simulink library "DLE_position_controller_v2"  (R2025b)
settings: Solver=VariableStepAuto  StartTime=0.0  StopTime=10.0  RelTol=1e-3
libraries: simulink x4, slpidlib x3, eeGeneralControl x1, dspstat3 x1
settings Model: Creator=cmmcguir  LastModifiedBy=cmmcguir

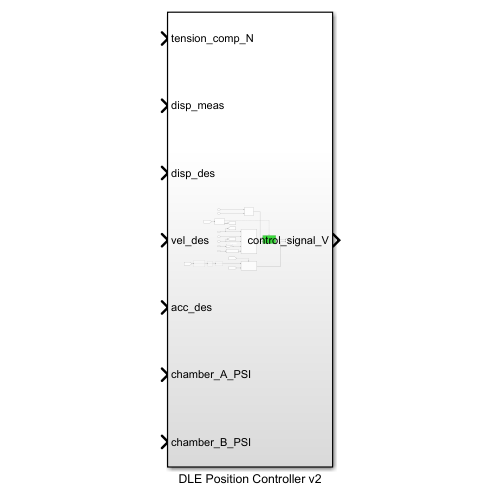
[thumbnail: Simulink's stored preview of the top-level diagram]
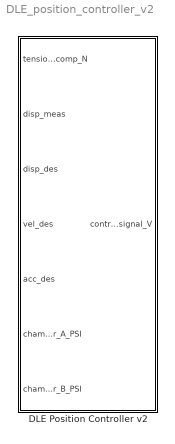
== system DLE_position_controller_v2 ==
  DLE Position Controller v2 : Subsystem

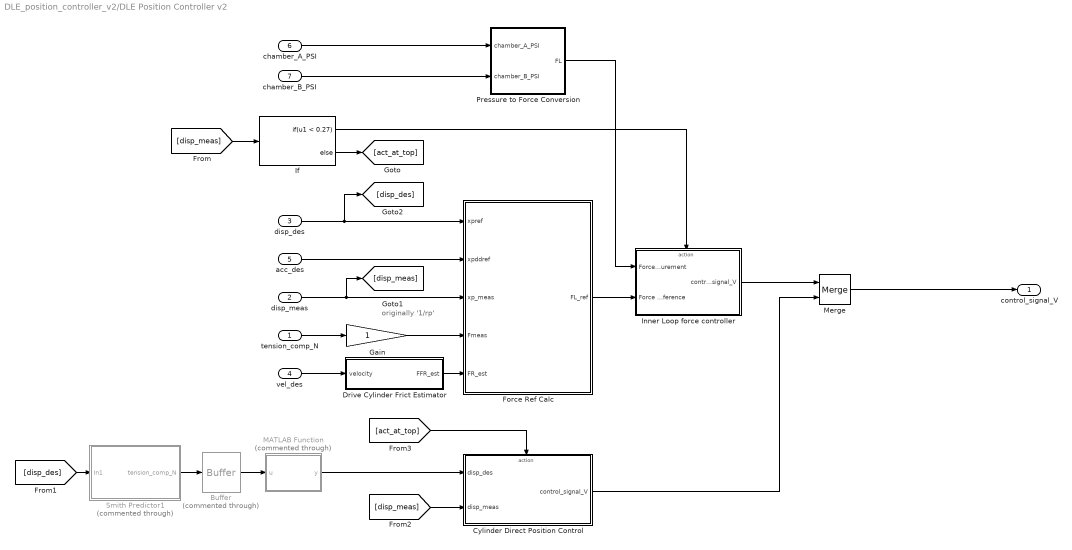
== system DLE_position_controller_v2/DLE Position Controller v2 ==
  note: originally '1/rp'
  tension_comp_N : Inport
  disp_meas : Inport  Port=2
  disp_des : Inport  Port=3
  vel_des : Inport  Port=4
  acc_des : Inport  Port=5
  chamber_A_PSI : Inport  Port=6
  chamber_B_PSI : Inport  Port=7
  Buffer : Buffer  Commented=through  OutputFrames=off
  Cylinder Direct Position Control : Subsystem  TreatAsAtomicUnit=on
  Drive Cylinder Frict Estimator : Subsystem
  Force Ref Calc : Subsystem
  Gain : Gain
  If : If  IfExpression=u1 < 0.27
  Inner Loop force controller : Subsystem  TreatAsAtomicUnit=on
  MATLAB Function : MATLAB Function  Commented=through  TreatAsAtomicUnit=on
  Merge : Merge
  Pressure to Force Conversion : Subsystem
  Smith Predictor1 : Subsystem  Commented=through
  control_signal_V : Outport
  wires:
  vel_des/1 -> Drive Cylinder Frict Estimator/1(velocity)
  disp_des/1 -> [disp_des], Force Ref Calc/1(xpref)
  acc_des/1 -> Force Ref Calc/2(xpddref)
  disp_meas/1 -> [disp_meas], Force Ref Calc/3(xp_meas)
  tension_comp_N/1 -> Gain/1
  Drive Cylinder Frict Estimator/1(FFR_est) -> Force Ref Calc/5(FR_est)
  chamber_A_PSI/1 -> Pressure to Force Conversion/1(chamber_A_PSI)
  chamber_B_PSI/1 -> Pressure to Force Conversion/2(chamber_B_PSI)
  Inner Loop force controller/1(control_signal_V) -> Merge/1
  Pressure to Force Conversion/1(FL) -> Inner Loop force controller/1(Force measurement)
  Force Ref Calc/1(FL_ref) -> Inner Loop force controller/2(Force reference)
  Gain/1 -> Force Ref Calc/4(Fmeas)
  If/1 -> Inner Loop force controller/Action
  If/2 -> [act_at_top]
  [disp_meas] -> If/1
  [disp_meas] -> Cylinder Direct Position Control/2(disp_meas)
  [act_at_top] -> Cylinder Direct Position Control/Action
  [disp_des] -> Smith Predictor1/1(In1)
  Cylinder Direct Position Control/1(control_signal_V) -> Merge/2
  Merge/1 -> control_signal_V/1
  MATLAB Function/1(y) -> Cylinder Direct Position Control/1(disp_des)
  Smith Predictor1/1(tension_comp_N) -> Buffer/1
  Buffer/1 -> MATLAB Function/1(u)

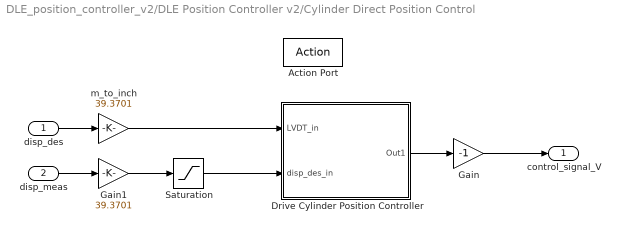
== system DLE_position_controller_v2/DLE Position Controller v2/Cylinder Direct Position Control ==
  disp_des : Inport
  disp_meas : Inport  Port=2
  Action Port : ActionPort
  Drive Cylinder Position Controller : Subsystem
  Gain : Gain  Gain=-1
  Gain1 : Gain  Gain=39.3701
  Saturation : Saturate  UpperLimit=12  LowerLimit=0
  m_to_inch : Gain  Gain=39.3701
  control_signal_V : Outport  VectorParamsAs1DForOutWhenUnconnected=off
  wires:
  Drive Cylinder Position Controller/1(Out1) -> Gain/1
  disp_des/1 -> m_to_inch/1
  Saturation/1 -> Drive Cylinder Position Controller/2(disp_des_in)
  disp_meas/1 -> Gain1/1
  Gain1/1 -> Saturation/1
  Gain/1 -> control_signal_V/1
  m_to_inch/1 -> Drive Cylinder Position Controller/1(LVDT_in)

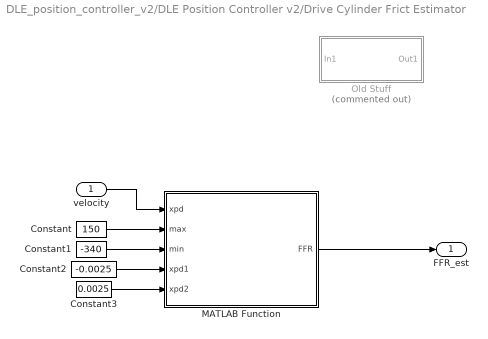
== system DLE_position_controller_v2/DLE Position Controller v2/Drive Cylinder Frict Estimator ==
  velocity : Inport
  Constant : Constant  Value=150
  Constant1 : Constant  Value=-340
  Constant2 : Constant  Value=-0.0025
  Constant3 : Constant  Value=0.0025
  MATLAB Function : MATLAB Function  TreatAsAtomicUnit=on
  Old Stuff : Subsystem  Commented=on
  FFR_est : Outport  VectorParamsAs1DForOutWhenUnconnected=off
  wires:
  velocity/1 -> MATLAB Function/1(xpd)
  Constant/1 -> MATLAB Function/2(max)
  Constant1/1 -> MATLAB Function/3(min)
  Constant2/1 -> MATLAB Function/4(xpd1)
  Constant3/1 -> MATLAB Function/5(xpd2)
  MATLAB Function/1(FFR) -> FFR_est/1

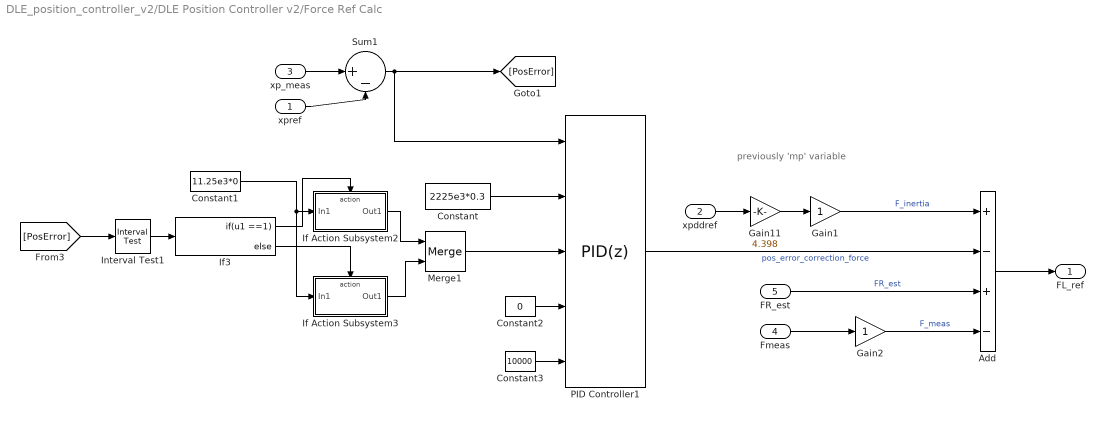
== system DLE_position_controller_v2/DLE Position Controller v2/Force Ref Calc ==
  note: previously 'mp' variable
  xpref : Inport
  xpddref : Inport  Port=2
  xp_meas : Inport  Port=3
  Fmeas : Inport  Port=4
  FR_est : Inport  Port=5
  " PID Controller1" : slpidlib/PID Controller  Controller=PID  Form=Parallel  TimeDomain=Discrete-time  UseExternalTs=off  SampleTime=-1  IntegratorMethod=Forward Euler  FilterMethod=Forward Euler  ControllerParametersSource=external  P=0.005  I=0.025  UseKiTs=off  D=0.001*0  UseExternalDerivativeSource=off  N=0.001  UseFilter=on  TunerSelectOption=Transfer Function Based (PID Tuner App)  InitialConditionSource=internal  InitialConditionForIntegrator=0  InitialConditionForFilter=0  DifferentiatorICPrevScaledInput=0  ExternalReset=none  TrackingMode=off  Kt=1  LimitOutput=on  SatLimitsSource=internal  UpperSaturationLimit=1000  LowerSaturationLimit=-1000  LinearizeAsGain=off  AntiWindupMode=clamping  Kb=1  LimitIntegrator=off  UpperIntegratorSaturationLimit=inf  LowerIntegratorSaturationLimit=-inf  POutMin=[]  POutMax=[]  IOutMin=[]  IOutMax=[]  DOutMin=[]  DOutMax=[]  NOutMin=[]  NOutMax=[]  SumOutMin=[]  SumOutMax=[]  SaturationOutMin=[]  SaturationOutMax=[]  PParamMin=[]  PParamMax=[]  IParamMin=[]  IParamMax=[]  DParamMin=[]  DParamMax=[]  NParamMin=[]  NParamMax=[]  KbParamMin=[]  KbParamMax=[]  KtParamMin=[]  KtParamMax=[]  KbOutMin=[]  KbOutMax=[]  KtOutMin=[]  KtOutMax=[]  IntegratorOutMin=[]  IntegratorOutMax=[]  FilterOutMin=[]  FilterOutMax=[]  SumI1OutMin=[]  SumI1OutMax=[]  SumI2OutMin=[]  SumI2OutMax=[]  SumI3OutMin=[]  SumI3OutMax=[]  SumI4OutMin=[]  SumI4OutMax=[]  SumDOutMin=[]  SumDOutMax=[]  DifferentiatorOutMin=[]  DifferentiatorOutMax=[]  FilterDiffOutCoefMin=[]  FilterDiffOutCoefMax=[]  ReciprocalOutMin=[]  ReciprocalOutMax=[]  SumDenOutMin=[]  SumDenOutMax=[]  SumNumOutMin=[]  SumNumOutMax=[]  DivideOutMin=[]  DivideOutMax=[]  UdiffTsProdOutMin=[]  UdiffTsProdOutMax=[]  NTsProdOutMin=[]  NTsProdOutMax=[]  UintegralTsProdOutMin=[]  UintegralTsProdOutMax=[]  UngainTsProdOutMin=[]  UngainTsProdOutMax=[]  ClampingZeroOutDataTypeStr=Inherit: Inherit via back propagation  ClampingZeroOutMin=[]  ClampingZeroOutMax=[]  FilterDenConstantOutDataTypeStr=Inherit: Inherit via back propagation  FilterDenConstantOutMin=[]  FilterDenConstantOutMax=[]  PCopyOutDataTypeStr=Inherit: Inherit via back propagation  PCopyOutMin=[]  PCopyOutMax=[]  NCopyOutDataTypeStr=Inherit: Inherit via back propagation  NCopyOutMin=[]  NCopyOutMax=[]  IntegratorContinuousStateAttributes=''  IntegratorStateMustResolveToSignalObject=off  IntegratorRTWStateStorageClass=Auto  FilterContinuousStateAttributes=''  FilterStateMustResolveToSignalObject=off  FilterRTWStateStorageClass=Auto  ParallelPVariant=ExternalParameters  IdealPVariant=Disabled  IVariant=ExternalParameters  DVariant=ExternalParameters  IntegratorVariant=Discrete  SatVariant=Enabled  AWVariant=DiscClampingParallel  PCopyVariant=Disabled  TRVariant=Disabled  FdbkBlocksVariant=Forward  IdealPFdbkVariant=Disabled  SatFdbkVariant=Disabled  DerivativeFilterVariant=ForwardEulerFilter  NVariant=ExternalParameters  NCopyVariant=Disabled  FilterICVariant=InternalICsFilter  IntegratorICVariant=InternalICs  ExternalResetVariant=Disabled  TRSumVariant=Passthrough  SumFdbkVariant=Disabled  SumVariant=Sum_PID  TsampFilterVariant=InternalTs  TsampNgainVariant=Passthrough  TsampIntegralVariant=Disabled_SignalSpec  ExternalSaturationOutDataTypeStr=Inherit: Same as second input  DerivativeSourceVariant=ErrorSignal  PreIntVariant=InternalPreInt
  Add : Sum  Inputs=+-+-
  Constant : Constant  Value=2225e3*0.3
  Constant1 : Constant  Value=11.25e3*0
  Constant2 : Constant  Value=0
  Constant3 : Constant  Value=10000
  Gain1 : Gain
  Gain11 : Gain  Gain=4.398
  Gain2 : Gain
  If Action Subsystem2 : Subsystem  TreatAsAtomicUnit=on
  If Action Subsystem3 : Subsystem  TreatAsAtomicUnit=on
  If3 : If  IfExpression=u1 ==1
  Interval Test1 : simulink/Logic and Bit Operations/Interval Test  IntervalClosedRight=on  uplimit=0  IntervalClosedLeft=on  lowlimit=0  OutDataTypeStr=boolean
  Merge1 : Merge
  Sum1 : Sum  Inputs=|+-
  FL_ref : Outport  VectorParamsAs1DForOutWhenUnconnected=off
  wires:
  xpddref/1 -> Gain11/1
  Gain11/1 -> Gain1/1
  Fmeas/1 -> Gain2/1
  Gain1/1 -> Add/1  "F_inertia"
  Gain2/1 -> Add/4  "F_meas"
  Constant2/1 -> " PID Controller1"/4
  Constant3/1 -> " PID Controller1"/5
  Constant/1 -> " PID Controller1"/2
  Sum1/1 -> [PosError], " PID Controller1"/1
  xp_meas/1 -> Sum1/1
  xpref/1 -> Sum1/2
  " PID Controller1"/1 -> Add/2  "pos_error_correction_force"
  If Action Subsystem2/1(Out1) -> Merge1/1
  If Action Subsystem3/1(Out1) -> Merge1/2
  [PosError] -> Interval Test1/1
  Interval Test1/1 -> If3/1
  Merge1/1 -> " PID Controller1"/3
  If3/1 -> If Action Subsystem2/Action
  Constant1/1 -> If Action Subsystem3/1(In1), If Action Subsystem2/1(In1)
  If3/2 -> If Action Subsystem3/Action
  FR_est/1 -> Add/3  "FR_est"
  Add/1 -> FL_ref/1

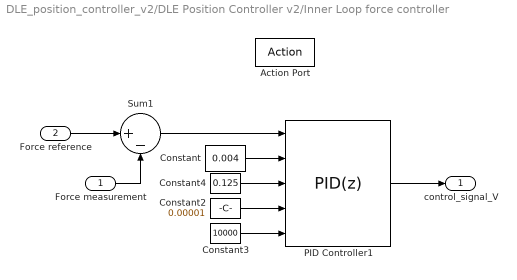
== system DLE_position_controller_v2/DLE Position Controller v2/Inner Loop force controller ==
  Force measurement : Inport
  Force reference : Inport  Port=2
  Action Port : ActionPort
  " PID Controller1" : slpidlib/PID Controller  Controller=PID  Form=Parallel  TimeDomain=Discrete-time  UseExternalTs=off  SampleTime=-1  IntegratorMethod=Forward Euler  FilterMethod=Forward Euler  ControllerParametersSource=external  P=0.005  I=0.025  UseKiTs=off  D=0.001*0  UseExternalDerivativeSource=off  N=0.001  UseFilter=on  TunerSelectOption=Transfer Function Based (PID Tuner App)  InitialConditionSource=internal  InitialConditionForIntegrator=0  InitialConditionForFilter=0  DifferentiatorICPrevScaledInput=0  ExternalReset=none  TrackingMode=off  Kt=1  LimitOutput=on  SatLimitsSource=internal  UpperSaturationLimit=10  LowerSaturationLimit=-10  LinearizeAsGain=off  AntiWindupMode=clamping  Kb=500  LimitIntegrator=off  UpperIntegratorSaturationLimit=inf  LowerIntegratorSaturationLimit=-inf  POutMin=[]  POutMax=[]  IOutMin=[]  IOutMax=[]  DOutMin=[]  DOutMax=[]  NOutMin=[]  NOutMax=[]  SumOutMin=[]  SumOutMax=[]  SaturationOutMin=[]  SaturationOutMax=[]  PParamMin=[]  PParamMax=[]  IParamMin=[]  IParamMax=[]  DParamMin=[]  DParamMax=[]  NParamMin=[]  NParamMax=[]  KbParamMin=[]  KbParamMax=[]  KtParamMin=[]  KtParamMax=[]  KbOutMin=[]  KbOutMax=[]  KtOutMin=[]  KtOutMax=[]  IntegratorOutMin=[]  IntegratorOutMax=[]  FilterOutMin=[]  FilterOutMax=[]  SumI1OutMin=[]  SumI1OutMax=[]  SumI2OutMin=[]  SumI2OutMax=[]  SumI3OutMin=[]  SumI3OutMax=[]  SumI4OutMin=[]  SumI4OutMax=[]  SumDOutMin=[]  SumDOutMax=[]  DifferentiatorOutMin=[]  DifferentiatorOutMax=[]  FilterDiffOutCoefMin=[]  FilterDiffOutCoefMax=[]  ReciprocalOutMin=[]  ReciprocalOutMax=[]  SumDenOutMin=[]  SumDenOutMax=[]  SumNumOutMin=[]  SumNumOutMax=[]  DivideOutMin=[]  DivideOutMax=[]  UdiffTsProdOutMin=[]  UdiffTsProdOutMax=[]  NTsProdOutMin=[]  NTsProdOutMax=[]  UintegralTsProdOutMin=[]  UintegralTsProdOutMax=[]  UngainTsProdOutMin=[]  UngainTsProdOutMax=[]  ClampingZeroOutDataTypeStr=Inherit: Inherit via back propagation  ClampingZeroOutMin=[]  ClampingZeroOutMax=[]  FilterDenConstantOutDataTypeStr=Inherit: Inherit via back propagation  FilterDenConstantOutMin=[]  FilterDenConstantOutMax=[]  PCopyOutDataTypeStr=Inherit: Inherit via back propagation  PCopyOutMin=[]  PCopyOutMax=[]  NCopyOutDataTypeStr=Inherit: Inherit via back propagation  NCopyOutMin=[]  NCopyOutMax=[]  IntegratorContinuousStateAttributes=''  IntegratorStateMustResolveToSignalObject=off  IntegratorRTWStateStorageClass=Auto  FilterContinuousStateAttributes=''  FilterStateMustResolveToSignalObject=off  FilterRTWStateStorageClass=Auto  ParallelPVariant=ExternalParameters  IdealPVariant=Disabled  IVariant=ExternalParameters  DVariant=ExternalParameters  IntegratorVariant=Discrete  SatVariant=Enabled  AWVariant=DiscClampingParallel  PCopyVariant=Disabled  TRVariant=Disabled  FdbkBlocksVariant=Forward  IdealPFdbkVariant=Disabled  SatFdbkVariant=Disabled  DerivativeFilterVariant=ForwardEulerFilter  NVariant=ExternalParameters  NCopyVariant=Disabled  FilterICVariant=InternalICsFilter  IntegratorICVariant=InternalICs  ExternalResetVariant=Disabled  TRSumVariant=Passthrough  SumFdbkVariant=Disabled  SumVariant=Sum_PID  TsampFilterVariant=InternalTs  TsampNgainVariant=Passthrough  TsampIntegralVariant=Disabled_SignalSpec  ExternalSaturationOutDataTypeStr=Inherit: Same as second input  DerivativeSourceVariant=ErrorSignal  PreIntVariant=InternalPreInt
  Constant : Constant  Value=0.004
  Constant2 : Constant  Value=0.00001
  Constant3 : Constant  Value=10000
  Constant4 : Constant  Value=0.125
  Sum1 : Sum  Inputs=|+-
  control_signal_V : Outport  VectorParamsAs1DForOutWhenUnconnected=off
  wires:
  Sum1/1 -> " PID Controller1"/1
  Force measurement/1 -> Sum1/2
  " PID Controller1"/1 -> control_signal_V/1
  Constant/1 -> " PID Controller1"/2
  Constant2/1 -> " PID Controller1"/4
  Constant3/1 -> " PID Controller1"/5
  Constant4/1 -> " PID Controller1"/3
  Force reference/1 -> Sum1/1

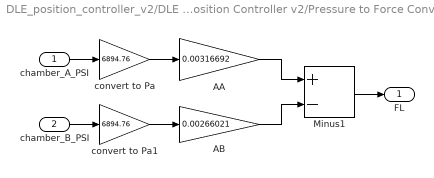
== system DLE_position_controller_v2/DLE Position Controller v2/Pressure to Force Conversion ==
  chamber_A_PSI : Inport
  chamber_B_PSI : Inport  Port=2
  AA : Gain  Gain=0.00316692
  AB : Gain  Gain=0.00266021
  Minus1 : Sum  Inputs=+-
  convert to Pa : Gain  Gain=6894.76
  convert to Pa1 : Gain  Gain=6894.76
  FL : Outport  VectorParamsAs1DForOutWhenUnconnected=off
  wires:
  Minus1/1 -> FL/1
  convert to Pa/1 -> AA/1
  AA/1 -> Minus1/1
  convert to Pa1/1 -> AB/1
  AB/1 -> Minus1/2
  chamber_A_PSI/1 -> convert to Pa/1
  chamber_B_PSI/1 -> convert to Pa1/1

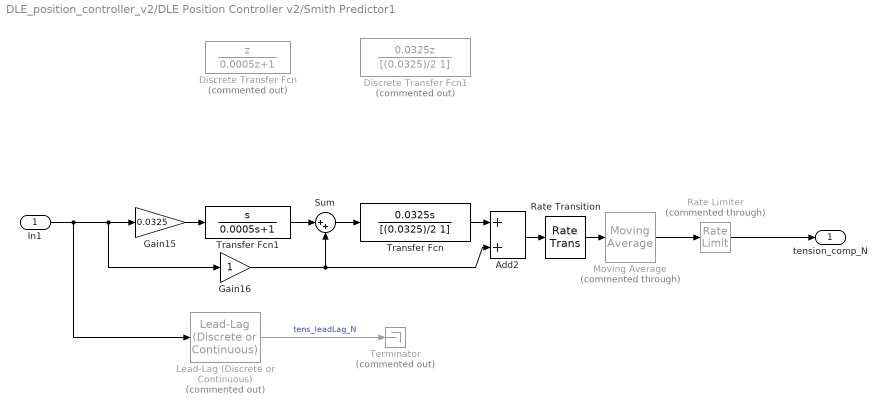
== system DLE_position_controller_v2/DLE Position Controller v2/Smith Predictor1 ==
  In1 : Inport
  Add2 : Sum
  Discrete Transfer Fcn : DiscreteTransferFcn  Commented=on  Numerator=[1 0]  Denominator=[0.0005 1]
  Discrete Transfer Fcn1 : DiscreteTransferFcn  Commented=on  Numerator=[0.0325 0]  Denominator=[(0.0325)/2 1]
  Gain15 : Gain  Gain=0.0325
  Gain16 : Gain
  Lead-Lag (Discrete or Continuous) : eeGeneralControl/Lead-Lag (Discrete or Continuous)  Commented=on  T1=0.3  T2=0.1  B=inf  A=-inf  init_option=Inherited from block input  x0=0  Ts=-1
  Moving Average : dspstat3/Moving Average  Commented=through  Method=Sliding window  ForgettingFactorPort=off  SpecifyWindowLength=on  WindowLength=50  OverlapLength=49  AllowArbitraryInputLength=off  ForgettingFactor=0.9  SimulateUsing=Interpreted execution
  Rate Limiter : RateLimiter  Commented=through  RisingSlewLimit=4e3  FallingSlewLimit=-4e3  SampleTimeMode=inherited
  Rate Transition : RateTransition  OutPortSampleTime=0.0001
  Sum : Sum  Inputs=|++
  Terminator : Terminator  Commented=on
  Transfer Fcn : TransferFcn  Numerator=[0.0325 0]  Denominator=[(0.0325)/2 1]
  Transfer Fcn1 : TransferFcn  Numerator=[1 0]  Denominator=[0.0005 1]
  tension_comp_N : Outport
  wires:
  Gain16/1 -> Sum/2, Add2/2
  Transfer Fcn1/1 -> Sum/1
  In1/1 -> Lead-Lag (Discrete or Continuous)/1, Gain15/1, Gain16/1
  Gain15/1 -> Transfer Fcn1/1
  Add2/1 -> Rate Transition/1
  Sum/1 -> Transfer Fcn/1
  Transfer Fcn/1 -> Add2/1
  Moving Average/1 -> Rate Limiter/1
  Rate Transition/1 -> Moving Average/1
  Lead-Lag (Discrete or Continuous)/1 -> Terminator/1  "tens_leadLag_N"
  Rate Limiter/1 -> tension_comp_N/1

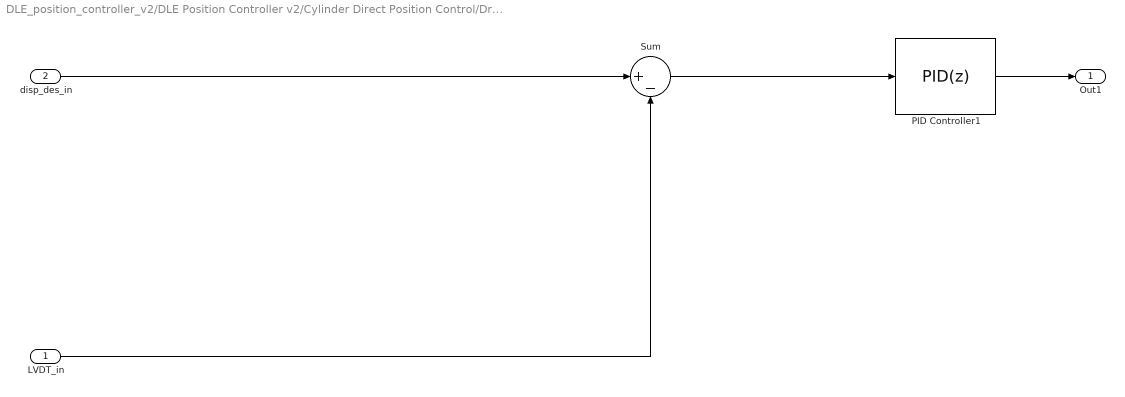
== system DLE_position_controller_v2/DLE Position Controller v2/Cylinder Direct Position Control/Drive Cylinder Position Controller ==
  LVDT_in : Inport
  disp_des_in : Inport  Port=2
  " PID Controller1" : slpidlib/PID Controller  Controller=PID  Form=Parallel  TimeDomain=Discrete-time  UseExternalTs=off  SampleTime=-1  IntegratorMethod=Forward Euler  FilterMethod=Forward Euler  ControllerParametersSource=internal  P=30*1  I=10*1  UseKiTs=off  D=0.75*0.25  UseExternalDerivativeSource=off  N=100  UseFilter=on  TunerSelectOption=Transfer Function Based (PID Tuner App)  InitialConditionSource=internal  InitialConditionForIntegrator=0  InitialConditionForFilter=0  DifferentiatorICPrevScaledInput=0  ExternalReset=none  TrackingMode=off  Kt=1  LimitOutput=on  SatLimitsSource=internal  UpperSaturationLimit=10  LowerSaturationLimit=-10  LinearizeAsGain=off  AntiWindupMode=clamping  Kb=1  LimitIntegrator=off  UpperIntegratorSaturationLimit=inf  LowerIntegratorSaturationLimit=-inf  POutMin=[]  POutMax=[]  IOutMin=[]  IOutMax=[]  DOutMin=[]  DOutMax=[]  NOutMin=[]  NOutMax=[]  SumOutMin=[]  SumOutMax=[]  SaturationOutMin=[]  SaturationOutMax=[]  PParamMin=[]  PParamMax=[]  IParamMin=[]  IParamMax=[]  DParamMin=[]  DParamMax=[]  NParamMin=[]  NParamMax=[]  KbParamMin=[]  KbParamMax=[]  KtParamMin=[]  KtParamMax=[]  KbOutMin=[]  KbOutMax=[]  KtOutMin=[]  KtOutMax=[]  IntegratorOutMin=[]  IntegratorOutMax=[]  FilterOutMin=[]  FilterOutMax=[]  SumI1OutMin=[]  SumI1OutMax=[]  SumI2OutMin=[]  SumI2OutMax=[]  SumI3OutMin=[]  SumI3OutMax=[]  SumI4OutMin=[]  SumI4OutMax=[]  SumDOutMin=[]  SumDOutMax=[]  DifferentiatorOutMin=[]  DifferentiatorOutMax=[]  FilterDiffOutCoefMin=[]  FilterDiffOutCoefMax=[]  ReciprocalOutMin=[]  ReciprocalOutMax=[]  SumDenOutMin=[]  SumDenOutMax=[]  SumNumOutMin=[]  SumNumOutMax=[]  DivideOutMin=[]  DivideOutMax=[]  UdiffTsProdOutMin=[]  UdiffTsProdOutMax=[]  NTsProdOutMin=[]  NTsProdOutMax=[]  UintegralTsProdOutMin=[]  UintegralTsProdOutMax=[]  UngainTsProdOutMin=[]  UngainTsProdOutMax=[]  ClampingZeroOutDataTypeStr=Inherit: Inherit via back propagation  ClampingZeroOutMin=[]  ClampingZeroOutMax=[]  FilterDenConstantOutDataTypeStr=Inherit: Inherit via back propagation  FilterDenConstantOutMin=[]  FilterDenConstantOutMax=[]  PCopyOutDataTypeStr=Inherit: Inherit via back propagation  PCopyOutMin=[]  PCopyOutMax=[]  NCopyOutDataTypeStr=Inherit: Inherit via back propagation  NCopyOutMin=[]  NCopyOutMax=[]  IntegratorContinuousStateAttributes=''  IntegratorStateMustResolveToSignalObject=off  IntegratorRTWStateStorageClass=Auto  FilterContinuousStateAttributes=''  FilterStateMustResolveToSignalObject=off  FilterRTWStateStorageClass=Auto  ParallelPVariant=InternalParameters  IdealPVariant=Disabled  IVariant=InternalParameters  DVariant=InternalParameters  IntegratorVariant=Discrete  SatVariant=Enabled  AWVariant=DiscClampingParallel  PCopyVariant=Disabled  TRVariant=Disabled  FdbkBlocksVariant=Forward  IdealPFdbkVariant=Disabled  SatFdbkVariant=Disabled  DerivativeFilterVariant=ForwardEulerFilter  NVariant=InternalParameters  NCopyVariant=Disabled  FilterICVariant=InternalICsFilter  IntegratorICVariant=InternalICs  ExternalResetVariant=Disabled  TRSumVariant=Passthrough  SumFdbkVariant=Disabled  SumVariant=Sum_PID  TsampFilterVariant=InternalTs  TsampNgainVariant=Passthrough  TsampIntegralVariant=Disabled_SignalSpec  ExternalSaturationOutDataTypeStr=Inherit: Same as second input  DerivativeSourceVariant=ErrorSignal  PreIntVariant=InternalPreInt
  Sum : Sum  Inputs=|+-
  Out1 : Outport  VectorParamsAs1DForOutWhenUnconnected=off
  wires:
  Sum/1 -> " PID Controller1"/1
  LVDT_in/1 -> Sum/2
  " PID Controller1"/1 -> Out1/1
  disp_des_in/1 -> Sum/1

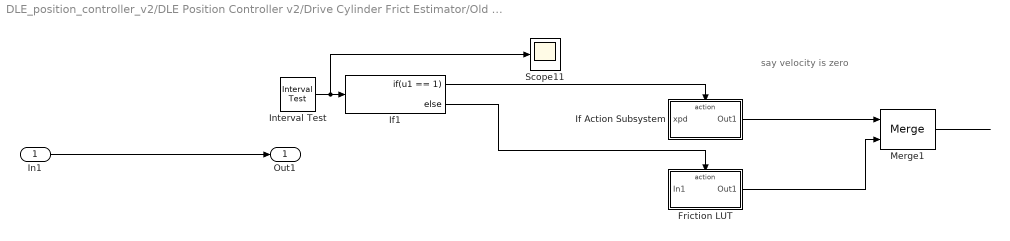
== system DLE_position_controller_v2/DLE Position Controller v2/Drive Cylinder Frict Estimator/Old Stuff ==
  note: say velocity is zero
  In1 : Inport
  Friction LUT : Subsystem  TreatAsAtomicUnit=on
  If Action Subsystem : Subsystem  TreatAsAtomicUnit=on
  If1 : If  IfExpression=u1 == 1
  Interval Test : simulink/Logic and Bit Operations/Interval Test  IntervalClosedRight=on  uplimit=0.006  IntervalClosedLeft=on  lowlimit=-0.004  OutDataTypeStr=boolean
  Merge1 : Merge
  Scope11 : Scope
      settings: ActiveDisplayYMinimum=-0.125  ActiveDisplayYMaximum=1.125
  Out1 : Outport  VectorParamsAs1DForOutWhenUnconnected=off
  wires:
  In1/1 -> Out1/1
  If1/2 -> Friction LUT/Action
  ? -> If Action Subsystem/1(xpd), Interval Test/1
  If1/1 -> If Action Subsystem/Action
  ? -> Friction LUT/1(In1)
  If Action Subsystem/1(Out1) -> Merge1/1
  Friction LUT/1(Out1) -> Merge1/2
  Interval Test/1 -> If1/1, Scope11/1
  Merge1/1 -> ?

== system DLE_position_controller_v2/DLE Position Controller v2/Force Ref Calc/If Action Subsystem2 ==
  In1 : Inport
  Action Port : ActionPort
  Gain : Gain  Gain=0
  Out1 : Outport  VectorParamsAs1DForOutWhenUnconnected=off
  wires:
  In1/1 -> Gain/1
  Gain/1 -> Out1/1

== system DLE_position_controller_v2/DLE Position Controller v2/Force Ref Calc/If Action Subsystem3 ==
  In1 : Inport
  Action Port : ActionPort
  Gain : Gain
  Out1 : Outport  VectorParamsAs1DForOutWhenUnconnected=off
  wires:
  In1/1 -> Gain/1
  Gain/1 -> Out1/1

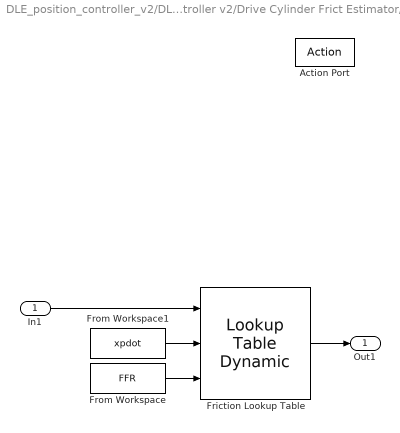
== system DLE_position_controller_v2/DLE Position Controller v2/Drive Cylinder Frict Estimator/Old Stuff/Friction LUT ==
  In1 : Inport
  Action Port : ActionPort
  Friction Lookup Table : simulink/Lookup Tables/Lookup Table Dynamic  LookUpMeth=Interpolation-Use End Values  OutDataType=fixdt('double')  OutScaling=[]  OutputDataTypeScalingMode=Specify via dialog  OutDataTypeStr=double  DoSatur=off
  From Workspace : FromWorkspace  VariableName=FFR
  From Workspace1 : FromWorkspace  VariableName=xpdot
  Out1 : Outport  VectorParamsAs1DForOutWhenUnconnected=off
  wires:
  From Workspace1/1 -> Friction Lookup Table/2
  From Workspace/1 -> Friction Lookup Table/3
  In1/1 -> Friction Lookup Table/1
  Friction Lookup Table/1 -> Out1/1

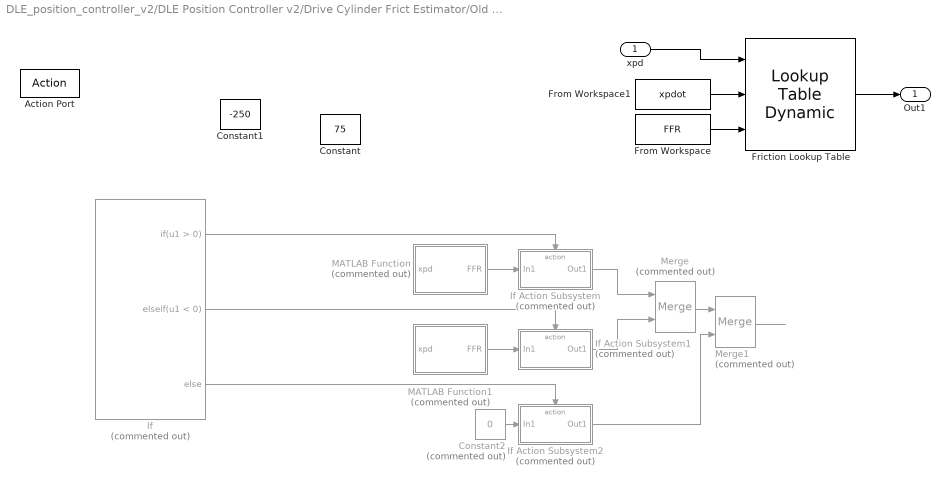
== system DLE_position_controller_v2/DLE Position Controller v2/Drive Cylinder Frict Estimator/Old Stuff/If Action Subsystem ==
  xpd : Inport
  Action Port : ActionPort
  Constant : Constant  Value=75
  Constant1 : Constant  Value=-250
  Constant2 : Constant  Commented=on  Value=0
  Friction Lookup Table : simulink/Lookup Tables/Lookup Table Dynamic  LookUpMeth=Interpolation-Use End Values  OutDataType=fixdt('double')  OutScaling=[]  OutputDataTypeScalingMode=Specify via dialog  OutDataTypeStr=double  DoSatur=off
  From Workspace : FromWorkspace  VariableName=FFR
  From Workspace1 : FromWorkspace  VariableName=xpdot
  If : If  Commented=on  ElseIfExpressions=u1 < 0
  If Action Subsystem : Subsystem  Commented=on  TreatAsAtomicUnit=on
  If Action Subsystem1 : Subsystem  Commented=on  TreatAsAtomicUnit=on
  If Action Subsystem2 : Subsystem  Commented=on  TreatAsAtomicUnit=on
  MATLAB Function : MATLAB Function  Commented=on  TreatAsAtomicUnit=on
  MATLAB Function1 : MATLAB Function  Commented=on  TreatAsAtomicUnit=on
  Merge : Merge  Commented=on
  Merge1 : Merge  Commented=on
  Out1 : Outport  VectorParamsAs1DForOutWhenUnconnected=off
  wires:
  Friction Lookup Table/1 -> Out1/1
  xpd/1 -> Friction Lookup Table/1
  From Workspace/1 -> Friction Lookup Table/3
  From Workspace1/1 -> Friction Lookup Table/2
  ? -> MATLAB Function/1(xpd), MATLAB Function1/1(xpd), If/1
  If Action Subsystem/1(Out1) -> Merge/1
  MATLAB Function/1(FFR) -> If Action Subsystem/1(In1)
  If/2 -> If Action Subsystem1/Action
  If Action Subsystem1/1(Out1) -> Merge/2
  If/1 -> If Action Subsystem/Action
  If/3 -> If Action Subsystem2/Action
  Merge/1 -> Merge1/1
  Merge1/1 -> ?
  If Action Subsystem2/1(Out1) -> Merge1/2
  Constant2/1 -> If Action Subsystem2/1(In1)
  MATLAB Function1/1(FFR) -> If Action Subsystem1/1(In1)

== system DLE_position_controller_v2/DLE Position Controller v2/Drive Cylinder Frict Estimator/Old Stuff/If Action Subsystem/If Action Subsystem ==
  In1 : Inport
  Action Port : ActionPort
  Out1 : Outport  VectorParamsAs1DForOutWhenUnconnected=off
  wires:
  In1/1 -> Out1/1

== system DLE_position_controller_v2/DLE Position Controller v2/Drive Cylinder Frict Estimator/Old Stuff/If Action Subsystem/If Action Subsystem1 ==
  In1 : Inport
  Action Port : ActionPort
  Out1 : Outport  VectorParamsAs1DForOutWhenUnconnected=off
  wires:
  In1/1 -> Out1/1

== system DLE_position_controller_v2/DLE Position Controller v2/Drive Cylinder Frict Estimator/Old Stuff/If Action Subsystem/If Action Subsystem2 ==
  In1 : Inport
  Action Port : ActionPort
  Out1 : Outport  VectorParamsAs1DForOutWhenUnconnected=off
  wires:
  In1/1 -> Out1/1

== matlab function DLE_position_controller_v2/DLE Position Controller v2/MATLAB Function ==
  data: u input; y output
function y = fcn(u)

[~, ind] = max(abs(u));
y = u(ind);

== matlab function DLE_position_controller_v2/DLE Position Controller v2/Drive Cylinder Frict Estimator/MATLAB Function ==
  data: xpd input; FFR output; max input; min input; xpd1 input; xpd2 input
function FFR = FrictionPoly(xpd, max, min,xpd1, xpd2)

p_pos = [286259495.429843,-173193752.694681,41175113.3821288,-4870042.97579715,308159.025845462,-8434.36139981410,146.161974739502];
p_neg = [-162371605.890866,-93401901.1521574,-21487354.7937511,-2556477.89021572,-183283.452954630,-6357.37685861595,-310.459473151221];


if xpd > xpd2
        
        if xpd <= 0.179334
            FFR = polyval(p_pos, xpd); %positive friction curve
        else
%             FFR = 3828.541*xpd - 249.1766; %linear extrapolation past what I have
                FFR = polyval(p_pos, .179334);
        end
    
elseif xpd < xpd1

        if xpd >= -0.1648
            FFR = polyval(p_neg, xpd); %negative friction curve
        else
%             FFR = 3211*xpd - 7.106;
                FFR = polyval(p_neg, -0.1648);
        end    
else
    

    FFR1 = polyval(p_neg, xpd1);
    FFR2 = polyval(p_pos, xpd2);

% FFR1 = min;
% FFR2 = max;
    
    FFR = interp1([xpd1 xpd2],[FFR1, FFR2], xpd);
% FFR = 0;
%     if xpdd > 0 %if concavity is positive
% %         
%        FFR = -350; %positive friction curve
% %        
%     elseif xpdd < 0
% % 
%         FFR = 150; %negative friction curve
%         
%     else
%         
%         FFR = 0;
%         
%     end

end

end

== matlab function DLE_position_controller_v2/DLE Position Controller v2/Drive Cylinder Frict Estimator/Old Stuff/If Action Subsystem/MATLAB Function ==
  data: xpd input; FFR output
function FFR = fcn(xpd)

FFR = 250/0.006*xpd; %linear fit for static friction force
end

== matlab function DLE_position_controller_v2/DLE Position Controller v2/Drive Cylinder Frict Estimator/Old Stuff/If Action Subsystem/MATLAB Function1 ==
  data: xpd input; FFR output
function FFR = fcn(xpd)

FFR = 450/0.004*xpd; %linear fit for static friction force
end
